simulink model "L1AC_test1_what_is_L1_adaptive"  (R2018b)
settings: Solver=ode14x  StartTime=0.0  StopTime=100  FixedStep=0.001  RelTol=1e-3
undefined symbols (not defined in the file or in its folder): kt, thet1o, thet2o
settings Model: Creator=Jcong  LastModifiedBy=Jcong

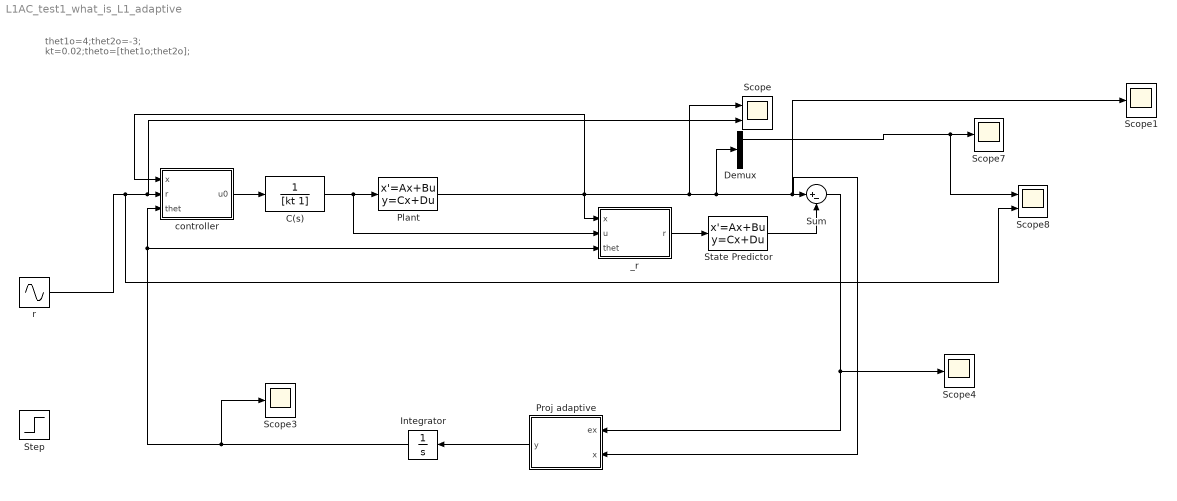
== system L1AC_test1_what_is_L1_adaptive ==
  note: thet1o=4;thet2o=-3;
      | kt=0.02;theto=[thet1o;thet2o];
  C(s) : TransferFcn  Denominator=[kt 1]
  Demux : Demux  Outputs=2
  Integrator : Integrator
  Plant : StateSpace  A=[0,1;(-0.3+thet1o),(-1+thet2o)]  B=[0;1]  C=[1,0;0,1]  D=[0;0]  InitialCondition=[1;1]
  Proj adaptive : MATLAB Function  TreatAsAtomicUnit=on
  Scope : Scope  NumInputPorts=2
  Scope{1,3..4,7} (4 alike) : Scope
  Scope8 : Scope  NumInputPorts=2
  State Predictor : StateSpace  A=[0,1;-0.3,-1]  B=[0;1]  C=[1,0;0,1]  D=[0;0]  InitialCondition=[1;1]
  Step : Step  SampleTime=0
  Sum : Sum  Inputs=|+-
  _r : MATLAB Function  TreatAsAtomicUnit=on
  controller : MATLAB Function  TreatAsAtomicUnit=on
  r : Sin  Amplitude=50  Frequency=0.5  SampleTime=0
  wires:
  _r/1(r) -> State Predictor/1
  Plant/1 -> Scope/1, Demux/1, Scope1/1, Proj adaptive/2(x), Sum/1, controller/1(x), _r/1(x)
  r/1 -> Scope8/2, Scope/2, controller/2(r)
  controller/1(u0) -> C(s)/1
  C(s)/1 -> _r/2(u), Plant/1
  State Predictor/1 -> Sum/2
  Sum/1 -> Scope4/1, Proj adaptive/1(ex)
  Proj adaptive/1(y) -> Integrator/1
  Integrator/1 -> Scope3/1, _r/3(thet), controller/3(thet)
  Demux/1 -> Scope8/1, Scope7/1

== matlab function L1AC_test1_what_is_L1_adaptive/controller ==
  data: x input; r input; u0 output; thet input
function u0 = fcn(x,r,thet)
k0=3/10;
u0 = -thet'*x+r*k0;

== matlab function L1AC_test1_what_is_L1_adaptive/_r ==
  data: x input; u input; r output; thet input
function r = fcn(x,u,thet)

r = thet'*x+u;

== matlab function L1AC_test1_what_is_L1_adaptive/Proj adaptive ==
  data: ex input; y output; x input
function y = fcn(ex,x)
b=[0;1];
T=10000;
P=500;
y =T*ex'*P*b*x;
